simulink model "Copy_of_nonlinear_model"  (R2021b)
settings: Solver=FixedStepAuto  StartTime=0.0  StopTime=RunTime  FixedStep=time_step  RelTol=1e-3
values from neighbouring files (symbols this model uses):
  init_theta_1 = pi    (= 3.14159265359)    [Copy_of_step2_whitebox_beam.m]    (also in compare_ourmodel_with_others.m = 0; linearize_script.m; step2_whitebox_beam.m; syms_test.m)
  init_theta_2 = pi/2    (= 1.57079632679)    [Copy_of_step2_whitebox_beam.m]    (also in compare_ourmodel_with_others.m = 0; linearize_script.m; step2_whitebox_beam.m = -1.57079632679; syms_test.m = 0)
settings Model: Creator=97083  LastModifiedBy=lyitingli
settings DataIOCC: ExternalInput=[u]
settings DebuggingCC: UnconnectedInputMsg=none  UnconnectedOutputMsg=none  UnconnectedLineMsg=none  UnderSpecifiedDimensionMsg=warning
settings ModelReferenceCC: EnableRefExpFcnMdlSchedulingChecks=off
settings RTWCC: DLArmComputeVersion=20.02.1

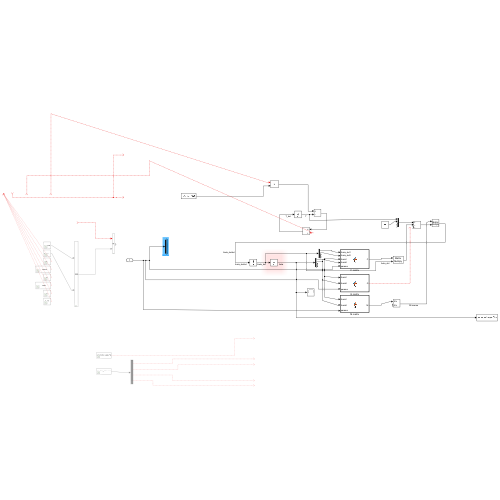
[thumbnail: Simulink's stored preview of the top-level diagram]
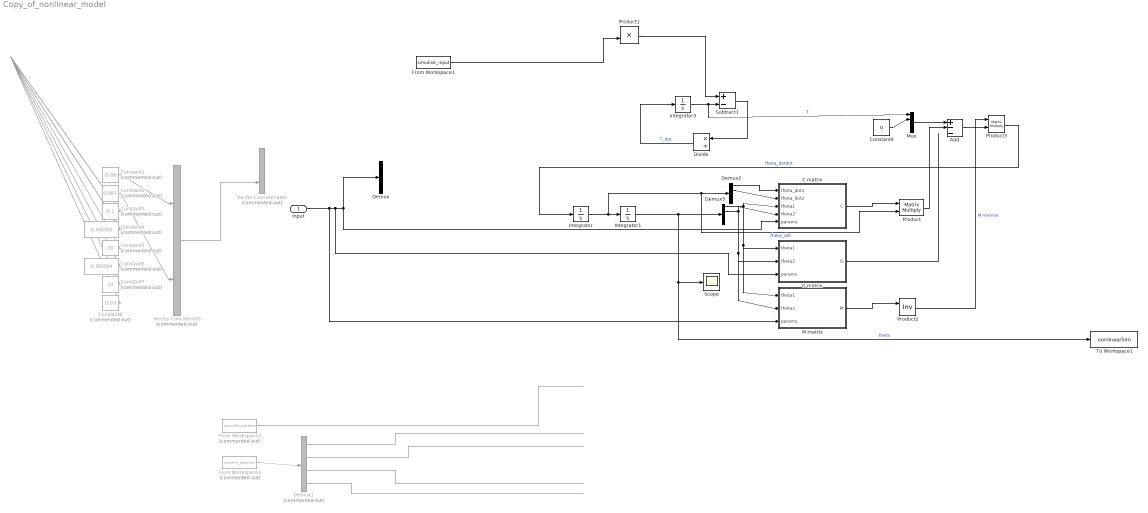
== system Copy_of_nonlinear_model ==
  Input : Inport
  Add : Sum  Inputs=+--
  C matrix : MATLAB Function  TreatAsAtomicUnit=on
  Constant1 : Constant  Commented=on  Value=-0.06
  Constant2 : Constant  Commented=on  Value=0.087
  Constant3 : Constant  Commented=on  Value=0.1
  Constant4 : Constant  Commented=on  Value=0.00004
  Constant5 : Constant  Commented=on  Value=30
  Constant6 : Constant  Commented=on  Value=0.00004
  Constant7 : Constant  Commented=on  Value=20
  Constant8 : Constant  Commented=on  Value=0.03
  Constant9 : Constant  Value=0
  Demux : Demux  Outputs=13
  Demux1 : Demux  Commented=on  Outputs=5
  Demux2 : Demux  Outputs=2
  Demux3 : Demux  Outputs=2
  Divide : Product  Inputs=*/
  From Workspace1 : FromWorkspace  SampleTime=-1
  From Workspace2 : FromWorkspace  Commented=on  VariableName=simulink_params  SampleTime=-1
  From Workspace3 : FromWorkspace  Commented=on  VariableName=simulink_params1  SampleTime=-1
  G matrix : MATLAB Function  TreatAsAtomicUnit=on
  Integrator : Integrator
  Integrator1 : Integrator  InitialCondition=[init_theta_1, init_theta_2]
  Integrator3 : Integrator
  M matrix : MATLAB Function  TreatAsAtomicUnit=on
  Mux : Mux  Inputs=2
  Product : Product  Inputs=**  Multiplication=Matrix(*)
  Product1 : Product  InputSameDT=on  RndMeth=Zero  SaturateOnIntegerOverflow=on  OutDataTypeStr=Inherit: Same as first input
  Product2 : Product  Inputs=/  Multiplication=Matrix(*)
  Product3 : Product  Inputs=**  Multiplication=Matrix(*)
  Scope : Scope
  Subtract1 : Sum  Inputs=+-
  To Workspace1 : ToWorkspace  VariableName=nonlinearSim  SampleTime=0.001
  Vector Concatenate : Concatenate  Commented=on  NumInputs=8
  Vector Concatenate1 : Concatenate  Commented=on
  wires:
  Constant1/1 -> Vector Concatenate/1
  Constant2/1 -> Vector Concatenate/2
  Constant3/1 -> ?
  Constant4/1 -> ?
  Constant5/1 -> ?
  Constant6/1 -> ?
  Constant7/1 -> ?
  Constant8/1 -> ?
  ? -> Vector Concatenate1/1
  Vector Concatenate/1 -> Vector Concatenate1/2
  G matrix/1(G) -> ?
  From Workspace1/1 -> Product1/2
  Product/1 -> Add/2
  Subtract1/1 -> Divide/1
  Add/1 -> Product3/2
  Demux2/1 -> C matrix/1(theta_dot1)
  Constant9/1 -> Mux/2
  Integrator3/1 -> Mux/1, Subtract1/2  "T"
  Divide/1 -> Integrator3/1  "T_dot"
  Demux3/1 -> M matrix/1(theta1), G matrix/1(theta1), C matrix/3(theta1)
  Product2/1 -> Product3/1  "M inverse"
  Product3/1 -> Integrator/1  "theta_dotdot"
  Product1/1 -> Subtract1/1
  Demux3/2 -> M matrix/2(theta2), G matrix/2(theta2), C matrix/4(theta2)
  M matrix/1(M) -> Product2/1
  Demux2/2 -> C matrix/2(theta_dot2)
  Integrator1/1 -> Demux3/1, To Workspace1/1, Scope/1  "theta"
  Mux/1 -> Add/1
  C matrix/1(C) -> Product/1
  Integrator/1 -> Product/2, Demux2/1, Integrator1/1  "theta_dot"
  Demux1/3 -> ?
  From Workspace3/1 -> Demux1/1
  Demux1/2 -> ?
  ? -> ?
  Demux1/4 -> ?
  From Workspace2/1 -> ?
  Demux1/1 -> ?
  ? -> Product1/1
  ? -> Divide/2
  Input/1 -> M matrix/3(params), G matrix/3(params), Demux/1, C matrix/5(params)

== matlab function Copy_of_nonlinear_model/C matrix ==
  data: theta_dot1 input; theta_dot2 input; theta1 input; theta2 input; C output; params input
function C = C(theta_dot1, theta_dot2, theta1, theta2, params)
l_1 = params(2);
m_2 = params(5);
P3 = m_2 * l_1 * params(7);

C00 = params(10) - P3 * theta_dot2 * sin(theta2);
C01 = -P3 * (theta_dot1 + theta_dot2) * sin(theta2);
C10 = P3 * theta_dot1 * sin(theta2);
C11 = params(11);

C = [C00 C01; C10 C11];

== matlab function Copy_of_nonlinear_model/G matrix ==
  data: theta1 input; theta2 input; G output; params input
function G = G(theta1, theta2, params)
g = params(1);
l_1 = params(2);
m_1 = params(4);
m_2 = params(5);

c_1_0 = params(6);
c_2_0 = params(7);

g1 = (m_1 * c_1_0 + m_2 * l_1) * g;
g2 = m_2 * c_2_0 * g;

G00 = -g1 * sin(theta1) - g2 * sin(theta1 + theta2);
G01 = -g2 * sin(theta1 + theta2);

G = [G00 G01];

== matlab function Copy_of_nonlinear_model/M matrix ==
  data: theta1 input; theta2 input; M output; params input
function M = M(theta1, theta2, params)
g = params(1);
l_1 = params(2);
m_1 = params(4);
m_2 = params(5);

c_1_0 = params(6);
c_2_0 = params(7);
I_1_0 = params(8);
I_2_0 = params(9);
P1 = m_1 * c_1_0 * c_1_0 + m_2 * l_1 * l_1 + I_1_0;
P2 = m_2 * c_2_0 * c_2_0 + I_2_0;
P3 = m_2 * l_1 * c_2_0;


M00 = P1 + P2 + 2 * P3 * cos(theta2);
M01 = P2 + P3 * cos(theta2);
M10 = M01;
M11 = P2;

M = [M00 M01; M10 M11];
